simulink model "modelo_diagrama_simulacion2"  (R2015a)
settings: Solver=ode45  StartTime=0.0  StopTime=10  RelTol=1e-3
undefined symbols (not defined in the file): G, Ts
settings Model: CovModelRefEnable=off  Creator=n221  LastModifiedBy=n221
settings DataIOCC: SaveFormat=Dataset
settings HardwareCC: ProdBitPerPointer=64  ProdLargestAtomicFloat=Float  ProdIntDivRoundTo=Zero  ProdEndianess=LittleEndian  ProdHWDeviceType=Specified
settings GRTTargetCC: GeneratePreprocessorConditionals=Use local settings

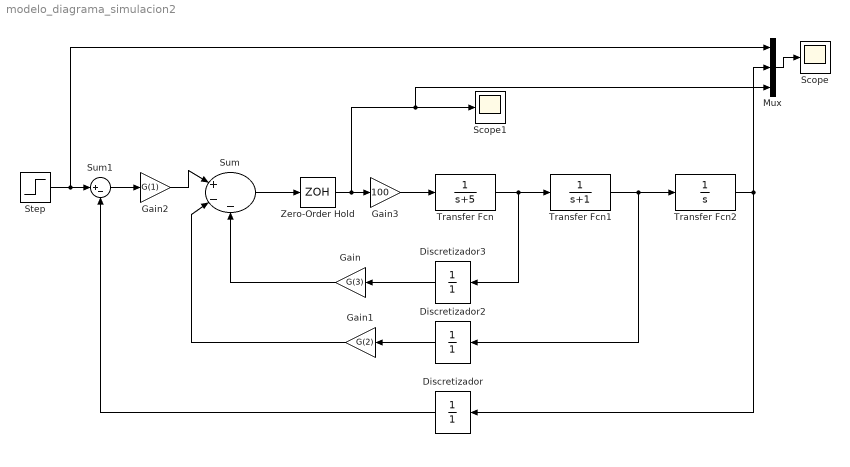
== system modelo_diagrama_simulacion2 ==
  " Discretizador2 " : DiscreteTransferFcn  Denominator=[1]  SampleTime=Ts
  " Discretizador3" : DiscreteTransferFcn  Denominator=[1]  SampleTime=Ts
  Discretizador : DiscreteTransferFcn  Denominator=[1]  SampleTime=Ts
  Gain : Gain  Gain=G(3)
  Gain1 : Gain  Gain=G(2)
  Gain2 : Gain  Gain=G(1)
  Gain3 : Gain  Gain=100
  Mux : Mux  Inputs=3
  Scope : Scope
      settings: TimeRange=auto  MaxDataPoints=5000  SaveName=datos  YMin=-0.19955  YMax=1.18155  SampleTime=-1
  Scope1 : Scope
      settings: TimeRange=auto  MaxDataPoints=5000  SaveToWorkspace=off  YMin=-0.13963  YMax=0.64227  SampleTime=-1
  Step : Step  Time=0  SampleTime=Ts
  Sum : Sum  Inputs=|+--
  Sum1 : Sum  Inputs=|+-
  Transfer Fcn : TransferFcn  Denominator=[1 5]
  Transfer Fcn1 : TransferFcn  Denominator=[1 1]
  Transfer Fcn2 : TransferFcn  Denominator=[1 0]
  Zero-Order Hold : ZeroOrderHold  SampleTime=Ts
  wires:
  Transfer Fcn1/1 -> " Discretizador2 "/1, Transfer Fcn2/1
  Transfer Fcn/1 -> " Discretizador3"/1, Transfer Fcn1/1
  Sum/1 -> Zero-Order Hold/1
  Step/1 -> Mux/1, Sum1/1
  Sum1/1 -> Gain2/1
  Transfer Fcn2/1 -> Discretizador/1, Mux/2
  Gain2/1 -> Sum/1
  Gain/1 -> Sum/3
  Gain1/1 -> Sum/2
  Zero-Order Hold/1 -> Mux/3, Scope1/1, Gain3/1
  Gain3/1 -> Transfer Fcn/1
  Mux/1 -> Scope/1
  " Discretizador3"/1 -> Gain/1
  " Discretizador2 "/1 -> Gain1/1
  Discretizador/1 -> Sum1/2
